simulink model "lab4_test2"  (R2016b)
settings: Solver=VariableStepAuto  StartTime=0.0  StopTime=totaltime  RelTol=1e-3
undefined symbols (not defined in the file or in its folder): h, st
libraries: xbsIndex_r4 x885
(part 2 of 2)

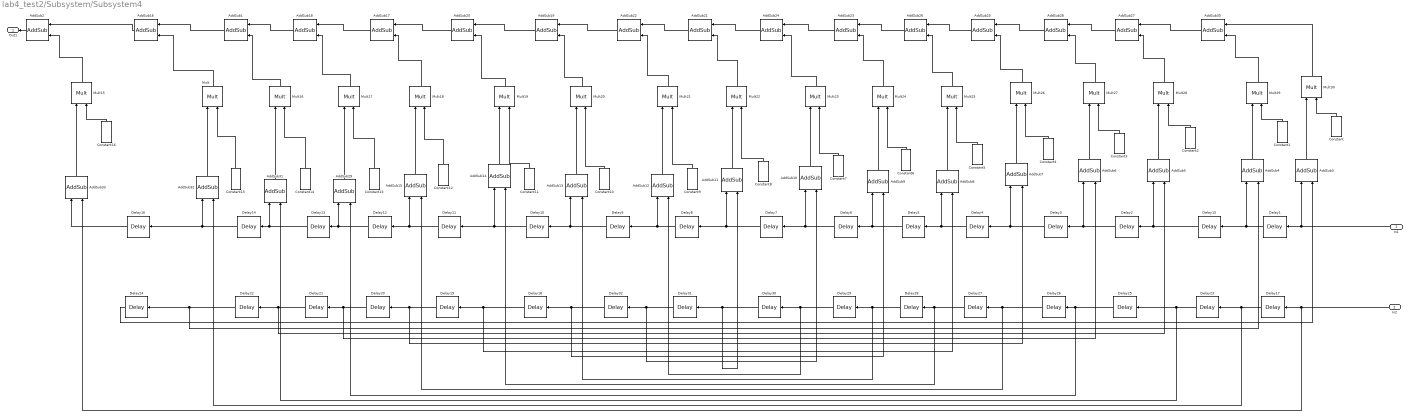
== system lab4_test2/Subsystem/Subsystem4 ==
  In1 : Inport
  In2 : Inport  Port=2
  AddSub{1..33} (33 alike) : xbsIndex_r4/AddSub  mode=Addition  use_carryin=off  use_carryout=off  en=off  latency=0  precision=User Defined  arith_type="Signed  (2's comp)"  n_bits=W  bin_pt=B  quantization=Truncate  overflow=Wrap  use_behavioral_HDL=off  hw_selection=Fabric  pipelined=off  dbl_ovrd=off  block_type=addsub
  Constant : xbsIndex_r4/Constant  const=h(1,10)  gui_display_data_type=Fixed-point  arith_type=Signed (2's comp)  n_bits=W  bin_pt=B  preci_type=Single  exp_width=8  frac_width=24  explicit_period=off  period=1  equ=P=C  opselect=C  inp2=PCIN>>17  opr=+  inp1=P  carry=CIN  dbl_ovrd=off  block_type=constant
  Constant1 : xbsIndex_r4/Constant  const=h(2,10)  gui_display_data_type=Fixed-point  arith_type=Signed (2's comp)  n_bits=W  bin_pt=B  preci_type=Single  exp_width=8  frac_width=24  explicit_period=off  period=1  equ=P=C  opselect=C  inp2=PCIN>>17  opr=+  inp1=P  carry=CIN  dbl_ovrd=off  block_type=constant
  Constant10 : xbsIndex_r4/Constant  const=h(11,10)  gui_display_data_type=Fixed-point  arith_type=Signed (2's comp)  n_bits=W  bin_pt=B  preci_type=Single  exp_width=8  frac_width=24  explicit_period=off  period=1  equ=P=C  opselect=C  inp2=PCIN>>17  opr=+  inp1=P  carry=CIN  dbl_ovrd=off  block_type=constant
  Constant11 : xbsIndex_r4/Constant  const=h(12,10)  gui_display_data_type=Fixed-point  arith_type=Signed (2's comp)  n_bits=W  bin_pt=B  preci_type=Single  exp_width=8  frac_width=24  explicit_period=off  period=1  equ=P=C  opselect=C  inp2=PCIN>>17  opr=+  inp1=P  carry=CIN  dbl_ovrd=off  block_type=constant
  Constant12 : xbsIndex_r4/Constant  const=h(13,10)  gui_display_data_type=Fixed-point  arith_type=Signed (2's comp)  n_bits=W  bin_pt=B  preci_type=Single  exp_width=8  frac_width=24  explicit_period=off  period=1  equ=P=C  opselect=C  inp2=PCIN>>17  opr=+  inp1=P  carry=CIN  dbl_ovrd=off  block_type=constant
  Constant13 : xbsIndex_r4/Constant  const=h(14,10)  gui_display_data_type=Fixed-point  arith_type=Signed (2's comp)  n_bits=W  bin_pt=B  preci_type=Single  exp_width=8  frac_width=24  explicit_period=off  period=1  equ=P=C  opselect=C  inp2=PCIN>>17  opr=+  inp1=P  carry=CIN  dbl_ovrd=off  block_type=constant
  Constant14 : xbsIndex_r4/Constant  const=h(15,10)  gui_display_data_type=Fixed-point  arith_type=Signed (2's comp)  n_bits=W  bin_pt=B  preci_type=Single  exp_width=8  frac_width=24  explicit_period=off  period=1  equ=P=C  opselect=C  inp2=PCIN>>17  opr=+  inp1=P  carry=CIN  dbl_ovrd=off  block_type=constant
  Constant15 : xbsIndex_r4/Constant  const=h(16,10)  gui_display_data_type=Fixed-point  arith_type=Signed (2's comp)  n_bits=W  bin_pt=B  preci_type=Single  exp_width=8  frac_width=24  explicit_period=off  period=1  equ=P=C  opselect=C  inp2=PCIN>>17  opr=+  inp1=P  carry=CIN  dbl_ovrd=off  block_type=constant
  Constant16 : xbsIndex_r4/Constant  const=h(17,10)  gui_display_data_type=Fixed-point  arith_type=Signed (2's comp)  n_bits=W  bin_pt=B  preci_type=Single  exp_width=8  frac_width=24  explicit_period=off  period=1  equ=P=C  opselect=C  inp2=PCIN>>17  opr=+  inp1=P  carry=CIN  dbl_ovrd=off  block_type=constant
  Constant2 : xbsIndex_r4/Constant  const=h(3,10)  gui_display_data_type=Fixed-point  arith_type=Signed (2's comp)  n_bits=W  bin_pt=B  preci_type=Single  exp_width=8  frac_width=24  explicit_period=off  period=1  equ=P=C  opselect=C  inp2=PCIN>>17  opr=+  inp1=P  carry=CIN  dbl_ovrd=off  block_type=constant
  Constant3 : xbsIndex_r4/Constant  const=h(4,10)  gui_display_data_type=Fixed-point  arith_type=Signed (2's comp)  n_bits=W  bin_pt=B  preci_type=Single  exp_width=8  frac_width=24  explicit_period=off  period=1  equ=P=C  opselect=C  inp2=PCIN>>17  opr=+  inp1=P  carry=CIN  dbl_ovrd=off  block_type=constant
  Constant4 : xbsIndex_r4/Constant  const=h(5,10)  gui_display_data_type=Fixed-point  arith_type=Signed (2's comp)  n_bits=W  bin_pt=B  preci_type=Single  exp_width=8  frac_width=24  explicit_period=off  period=1  equ=P=C  opselect=C  inp2=PCIN>>17  opr=+  inp1=P  carry=CIN  dbl_ovrd=off  block_type=constant
  Constant5 : xbsIndex_r4/Constant  const=h(6,10)  gui_display_data_type=Fixed-point  arith_type=Signed (2's comp)  n_bits=W  bin_pt=B  preci_type=Single  exp_width=8  frac_width=24  explicit_period=off  period=1  equ=P=C  opselect=C  inp2=PCIN>>17  opr=+  inp1=P  carry=CIN  dbl_ovrd=off  block_type=constant
  Constant6 : xbsIndex_r4/Constant  const=h(7,10)  gui_display_data_type=Fixed-point  arith_type=Signed (2's comp)  n_bits=W  bin_pt=B  preci_type=Single  exp_width=8  frac_width=24  explicit_period=off  period=1  equ=P=C  opselect=C  inp2=PCIN>>17  opr=+  inp1=P  carry=CIN  dbl_ovrd=off  block_type=constant
  Constant7 : xbsIndex_r4/Constant  const=h(8,10)  gui_display_data_type=Fixed-point  arith_type=Signed (2's comp)  n_bits=W  bin_pt=B  preci_type=Single  exp_width=8  frac_width=24  explicit_period=off  period=1  equ=P=C  opselect=C  inp2=PCIN>>17  opr=+  inp1=P  carry=CIN  dbl_ovrd=off  block_type=constant
  Constant8 : xbsIndex_r4/Constant  const=h(9,10)  gui_display_data_type=Fixed-point  arith_type=Signed (2's comp)  n_bits=W  bin_pt=B  preci_type=Single  exp_width=8  frac_width=24  explicit_period=off  period=1  equ=P=C  opselect=C  inp2=PCIN>>17  opr=+  inp1=P  carry=CIN  dbl_ovrd=off  block_type=constant
  Constant9 : xbsIndex_r4/Constant  const=h(10,10)  gui_display_data_type=Fixed-point  arith_type=Signed (2's comp)  n_bits=W  bin_pt=B  preci_type=Single  exp_width=8  frac_width=24  explicit_period=off  period=1  equ=P=C  opselect=C  inp2=PCIN>>17  opr=+  inp1=P  carry=CIN  dbl_ovrd=off  block_type=constant
  Delay{1..32} (32 alike) : xbsIndex_r4/Delay  rst=off  infoeditControl=Selection of Reset will increase slice count due to use of real FFs and instead of SRLs  en=off  latency=1  reg_retiming=off  dbl_ovrd=off  block_type=delay
  Mult{,15..30} (17 alike) : xbsIndex_r4/Mult  precision=User Defined  arith_type="Signed  (2's comp)"  n_bits=W  bin_pt=B  quantization="Round  (unbiased: +/- Inf)"  overflow=Flag as error  en=off  latency=0  use_behavioral_HDL=off  opt=Speed  use_embedded=on  optimum_pipeline=off  pipeline=on  dbl_ovrd=off  use_rpm=on  placement_style=Triangular  block_type=mult
  Out1 : Outport
  wires:
  AddSub2/1 -> Out1/1
  Constant14/1 -> Mult16/2
  Mult/1 -> AddSub16/2
  Mult16/1 -> AddSub1/2
  Constant15/1 -> Mult/2
  Constant13/1 -> Mult17/2
  Mult17/1 -> AddSub18/2
  Constant12/1 -> Mult18/2
  Constant11/1 -> Mult19/2
  Mult19/1 -> AddSub20/2
  Constant10/1 -> Mult20/2
  Mult20/1 -> AddSub19/2
  Constant9/1 -> Mult21/2
  Mult21/1 -> AddSub22/2
  Constant8/1 -> Mult22/2
  Constant7/1 -> Mult23/2
  Mult23/1 -> AddSub24/2
  Constant6/1 -> Mult24/2
  Constant5/1 -> Mult25/2
  Mult25/1 -> AddSub26/2
  Constant4/1 -> Mult26/2
  Mult26/1 -> AddSub25/2
  Constant3/1 -> Mult27/2
  Mult27/1 -> AddSub28/2
  Constant2/1 -> Mult28/2
  Constant1/1 -> Mult29/2
  Mult29/1 -> AddSub30/2
  Constant/1 -> Mult30/2
  AddSub1/1 -> AddSub16/1
  AddSub18/1 -> AddSub1/1
  AddSub17/1 -> AddSub18/1
  AddSub19/1 -> AddSub20/1
  AddSub22/1 -> AddSub19/1
  AddSub21/1 -> AddSub22/1
  AddSub23/1 -> AddSub24/1
  AddSub25/1 -> AddSub26/1
  AddSub28/1 -> AddSub25/1
  AddSub27/1 -> AddSub28/1
  Mult30/1 -> AddSub30/1
  Constant16/1 -> Mult15/2
  Mult15/1 -> AddSub2/2
  AddSub16/1 -> AddSub2/1
  AddSub20/1 -> AddSub17/1
  Mult18/1 -> AddSub17/2
  AddSub24/1 -> AddSub21/1
  Mult22/1 -> AddSub21/2
  AddSub26/1 -> AddSub23/1
  Mult24/1 -> AddSub23/2
  AddSub30/1 -> AddSub27/1
  Mult28/1 -> AddSub27/2
  In1/1 -> AddSub3/1, Delay1/1
  Delay1/1 -> AddSub4/1, Delay15/1
  Delay15/1 -> AddSub5/1, Delay2/1
  Delay2/1 -> AddSub6/1, Delay3/1
  Delay3/1 -> AddSub7/1, Delay4/1
  Delay4/1 -> AddSub8/1, Delay5/1
  Delay5/1 -> AddSub9/1, Delay6/1
  Delay6/1 -> AddSub10/1, Delay7/1
  Delay7/1 -> AddSub11/1, Delay8/1
  Delay8/1 -> AddSub12/1, Delay9/1
  Delay9/1 -> AddSub13/1, Delay10/1
  Delay10/1 -> AddSub14/1, Delay11/1
  Delay11/1 -> AddSub15/1, Delay12/1
  Delay12/1 -> AddSub29/1, Delay13/1
  Delay13/1 -> AddSub31/1, Delay14/1
  Delay14/1 -> AddSub32/1, Delay16/1
  In2/1 -> AddSub33/2, Delay17/1
  Delay17/1 -> AddSub32/2, Delay23/1
  Delay23/1 -> AddSub31/2, Delay25/1
  Delay25/1 -> AddSub29/2, Delay26/1
  Delay26/1 -> AddSub15/2, Delay27/1
  Delay27/1 -> AddSub14/2, Delay28/1
  Delay28/1 -> AddSub13/2, Delay29/1
  Delay29/1 -> AddSub12/2, Delay30/1
  Delay30/1 -> AddSub11/2, Delay31/1
  Delay31/1 -> AddSub10/2, Delay32/1
  Delay32/1 -> AddSub9/2, Delay18/1
  Delay18/1 -> AddSub8/2, Delay19/1
  Delay19/1 -> AddSub7/2, Delay20/1
  Delay20/1 -> AddSub6/2, Delay21/1
  Delay21/1 -> AddSub5/2, Delay22/1
  Delay22/1 -> AddSub4/2, Delay24/1
  AddSub3/1 -> Mult30/1
  Delay16/1 -> AddSub33/1
  AddSub33/1 -> Mult15/1
  AddSub32/1 -> Mult/1
  AddSub31/1 -> Mult16/1
  AddSub29/1 -> Mult17/1
  AddSub15/1 -> Mult18/1
  AddSub14/1 -> Mult19/1
  AddSub13/1 -> Mult20/1
  AddSub12/1 -> Mult21/1
  AddSub11/1 -> Mult22/1
  AddSub10/1 -> Mult23/1
  AddSub9/1 -> Mult24/1
  AddSub8/1 -> Mult25/1
  AddSub7/1 -> Mult26/1
  AddSub6/1 -> Mult27/1
  AddSub5/1 -> Mult28/1
  AddSub4/1 -> Mult29/1
  Delay24/1 -> AddSub3/2

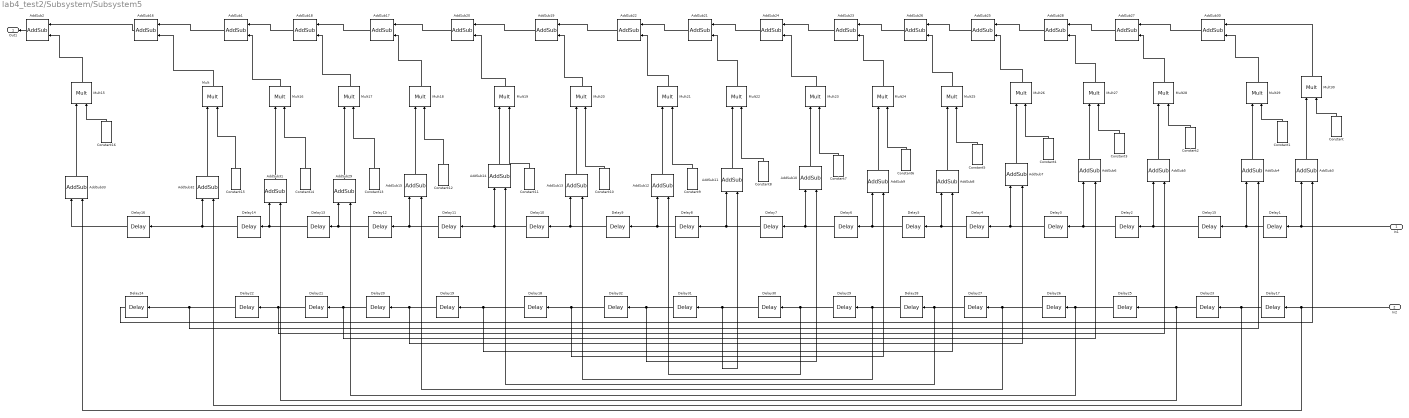
== system lab4_test2/Subsystem/Subsystem5 ==
  In1 : Inport
  In2 : Inport  Port=2
  AddSub{1..33} (33 alike) : xbsIndex_r4/AddSub  mode=Addition  use_carryin=off  use_carryout=off  en=off  latency=0  precision=User Defined  arith_type="Signed  (2's comp)"  n_bits=W  bin_pt=B  quantization=Truncate  overflow=Wrap  use_behavioral_HDL=off  hw_selection=Fabric  pipelined=off  dbl_ovrd=off  block_type=addsub
  Constant : xbsIndex_r4/Constant  const=h(1,13)  gui_display_data_type=Fixed-point  arith_type=Signed (2's comp)  n_bits=W  bin_pt=B  preci_type=Single  exp_width=8  frac_width=24  explicit_period=off  period=1  equ=P=C  opselect=C  inp2=PCIN>>17  opr=+  inp1=P  carry=CIN  dbl_ovrd=off  block_type=constant
  Constant1 : xbsIndex_r4/Constant  const=h(2,13)  gui_display_data_type=Fixed-point  arith_type=Signed (2's comp)  n_bits=W  bin_pt=B  preci_type=Single  exp_width=8  frac_width=24  explicit_period=off  period=1  equ=P=C  opselect=C  inp2=PCIN>>17  opr=+  inp1=P  carry=CIN  dbl_ovrd=off  block_type=constant
  Constant10 : xbsIndex_r4/Constant  const=h(11,13)  gui_display_data_type=Fixed-point  arith_type=Signed (2's comp)  n_bits=W  bin_pt=B  preci_type=Single  exp_width=8  frac_width=24  explicit_period=off  period=1  equ=P=C  opselect=C  inp2=PCIN>>17  opr=+  inp1=P  carry=CIN  dbl_ovrd=off  block_type=constant
  Constant11 : xbsIndex_r4/Constant  const=h(12,13)  gui_display_data_type=Fixed-point  arith_type=Signed (2's comp)  n_bits=W  bin_pt=B  preci_type=Single  exp_width=8  frac_width=24  explicit_period=off  period=1  equ=P=C  opselect=C  inp2=PCIN>>17  opr=+  inp1=P  carry=CIN  dbl_ovrd=off  block_type=constant
  Constant12 : xbsIndex_r4/Constant  const=h(13,13)  gui_display_data_type=Fixed-point  arith_type=Signed (2's comp)  n_bits=W  bin_pt=B  preci_type=Single  exp_width=8  frac_width=24  explicit_period=off  period=1  equ=P=C  opselect=C  inp2=PCIN>>17  opr=+  inp1=P  carry=CIN  dbl_ovrd=off  block_type=constant
  Constant13 : xbsIndex_r4/Constant  const=h(14,13)  gui_display_data_type=Fixed-point  arith_type=Signed (2's comp)  n_bits=W  bin_pt=B  preci_type=Single  exp_width=8  frac_width=24  explicit_period=off  period=1  equ=P=C  opselect=C  inp2=PCIN>>17  opr=+  inp1=P  carry=CIN  dbl_ovrd=off  block_type=constant
  Constant14 : xbsIndex_r4/Constant  const=h(15,13)  gui_display_data_type=Fixed-point  arith_type=Signed (2's comp)  n_bits=W  bin_pt=B  preci_type=Single  exp_width=8  frac_width=24  explicit_period=off  period=1  equ=P=C  opselect=C  inp2=PCIN>>17  opr=+  inp1=P  carry=CIN  dbl_ovrd=off  block_type=constant
  Constant15 : xbsIndex_r4/Constant  const=h(16,13)  gui_display_data_type=Fixed-point  arith_type=Signed (2's comp)  n_bits=W  bin_pt=B  preci_type=Single  exp_width=8  frac_width=24  explicit_period=off  period=1  equ=P=C  opselect=C  inp2=PCIN>>17  opr=+  inp1=P  carry=CIN  dbl_ovrd=off  block_type=constant
  Constant16 : xbsIndex_r4/Constant  const=h(17,13)  gui_display_data_type=Fixed-point  arith_type=Signed (2's comp)  n_bits=W  bin_pt=B  preci_type=Single  exp_width=8  frac_width=24  explicit_period=off  period=1  equ=P=C  opselect=C  inp2=PCIN>>17  opr=+  inp1=P  carry=CIN  dbl_ovrd=off  block_type=constant
  Constant2 : xbsIndex_r4/Constant  const=h(3,13)  gui_display_data_type=Fixed-point  arith_type=Signed (2's comp)  n_bits=W  bin_pt=B  preci_type=Single  exp_width=8  frac_width=24  explicit_period=off  period=1  equ=P=C  opselect=C  inp2=PCIN>>17  opr=+  inp1=P  carry=CIN  dbl_ovrd=off  block_type=constant
  Constant3 : xbsIndex_r4/Constant  const=h(4,13)  gui_display_data_type=Fixed-point  arith_type=Signed (2's comp)  n_bits=W  bin_pt=B  preci_type=Single  exp_width=8  frac_width=24  explicit_period=off  period=1  equ=P=C  opselect=C  inp2=PCIN>>17  opr=+  inp1=P  carry=CIN  dbl_ovrd=off  block_type=constant
  Constant4 : xbsIndex_r4/Constant  const=h(5,13)  gui_display_data_type=Fixed-point  arith_type=Signed (2's comp)  n_bits=W  bin_pt=B  preci_type=Single  exp_width=8  frac_width=24  explicit_period=off  period=1  equ=P=C  opselect=C  inp2=PCIN>>17  opr=+  inp1=P  carry=CIN  dbl_ovrd=off  block_type=constant
  Constant5 : xbsIndex_r4/Constant  const=h(6,13)  gui_display_data_type=Fixed-point  arith_type=Signed (2's comp)  n_bits=W  bin_pt=B  preci_type=Single  exp_width=8  frac_width=24  explicit_period=off  period=1  equ=P=C  opselect=C  inp2=PCIN>>17  opr=+  inp1=P  carry=CIN  dbl_ovrd=off  block_type=constant
  Constant6 : xbsIndex_r4/Constant  const=h(7,13)  gui_display_data_type=Fixed-point  arith_type=Signed (2's comp)  n_bits=W  bin_pt=B  preci_type=Single  exp_width=8  frac_width=24  explicit_period=off  period=1  equ=P=C  opselect=C  inp2=PCIN>>17  opr=+  inp1=P  carry=CIN  dbl_ovrd=off  block_type=constant
  Constant7 : xbsIndex_r4/Constant  const=h(8,13)  gui_display_data_type=Fixed-point  arith_type=Signed (2's comp)  n_bits=W  bin_pt=B  preci_type=Single  exp_width=8  frac_width=24  explicit_period=off  period=1  equ=P=C  opselect=C  inp2=PCIN>>17  opr=+  inp1=P  carry=CIN  dbl_ovrd=off  block_type=constant
  Constant8 : xbsIndex_r4/Constant  const=h(9,13)  gui_display_data_type=Fixed-point  arith_type=Signed (2's comp)  n_bits=W  bin_pt=B  preci_type=Single  exp_width=8  frac_width=24  explicit_period=off  period=1  equ=P=C  opselect=C  inp2=PCIN>>17  opr=+  inp1=P  carry=CIN  dbl_ovrd=off  block_type=constant
  Constant9 : xbsIndex_r4/Constant  const=h(10,13)  gui_display_data_type=Fixed-point  arith_type=Signed (2's comp)  n_bits=W  bin_pt=B  preci_type=Single  exp_width=8  frac_width=24  explicit_period=off  period=1  equ=P=C  opselect=C  inp2=PCIN>>17  opr=+  inp1=P  carry=CIN  dbl_ovrd=off  block_type=constant
  Delay{1..32} (32 alike) : xbsIndex_r4/Delay  rst=off  infoeditControl=Selection of Reset will increase slice count due to use of real FFs and instead of SRLs  en=off  latency=1  reg_retiming=off  dbl_ovrd=off  block_type=delay
  Mult{,15..30} (17 alike) : xbsIndex_r4/Mult  precision=User Defined  arith_type="Signed  (2's comp)"  n_bits=W  bin_pt=B  quantization="Round  (unbiased: +/- Inf)"  overflow=Flag as error  en=off  latency=0  use_behavioral_HDL=off  opt=Speed  use_embedded=on  optimum_pipeline=off  pipeline=on  dbl_ovrd=off  use_rpm=on  placement_style=Triangular  block_type=mult
  Out1 : Outport
  wires:
  AddSub2/1 -> Out1/1
  Constant14/1 -> Mult16/2
  Mult/1 -> AddSub16/2
  Mult16/1 -> AddSub1/2
  Constant15/1 -> Mult/2
  Constant13/1 -> Mult17/2
  Mult17/1 -> AddSub18/2
  Constant12/1 -> Mult18/2
  Constant11/1 -> Mult19/2
  Mult19/1 -> AddSub20/2
  Constant10/1 -> Mult20/2
  Mult20/1 -> AddSub19/2
  Constant9/1 -> Mult21/2
  Mult21/1 -> AddSub22/2
  Constant8/1 -> Mult22/2
  Constant7/1 -> Mult23/2
  Mult23/1 -> AddSub24/2
  Constant6/1 -> Mult24/2
  Constant5/1 -> Mult25/2
  Mult25/1 -> AddSub26/2
  Constant4/1 -> Mult26/2
  Mult26/1 -> AddSub25/2
  Constant3/1 -> Mult27/2
  Mult27/1 -> AddSub28/2
  Constant2/1 -> Mult28/2
  Constant1/1 -> Mult29/2
  Mult29/1 -> AddSub30/2
  Constant/1 -> Mult30/2
  AddSub1/1 -> AddSub16/1
  AddSub18/1 -> AddSub1/1
  AddSub17/1 -> AddSub18/1
  AddSub19/1 -> AddSub20/1
  AddSub22/1 -> AddSub19/1
  AddSub21/1 -> AddSub22/1
  AddSub23/1 -> AddSub24/1
  AddSub25/1 -> AddSub26/1
  AddSub28/1 -> AddSub25/1
  AddSub27/1 -> AddSub28/1
  Mult30/1 -> AddSub30/1
  Constant16/1 -> Mult15/2
  Mult15/1 -> AddSub2/2
  AddSub16/1 -> AddSub2/1
  AddSub20/1 -> AddSub17/1
  Mult18/1 -> AddSub17/2
  AddSub24/1 -> AddSub21/1
  Mult22/1 -> AddSub21/2
  AddSub26/1 -> AddSub23/1
  Mult24/1 -> AddSub23/2
  AddSub30/1 -> AddSub27/1
  Mult28/1 -> AddSub27/2
  In1/1 -> AddSub3/1, Delay1/1
  Delay1/1 -> AddSub4/1, Delay15/1
  Delay15/1 -> AddSub5/1, Delay2/1
  Delay2/1 -> AddSub6/1, Delay3/1
  Delay3/1 -> AddSub7/1, Delay4/1
  Delay4/1 -> AddSub8/1, Delay5/1
  Delay5/1 -> AddSub9/1, Delay6/1
  Delay6/1 -> AddSub10/1, Delay7/1
  Delay7/1 -> AddSub11/1, Delay8/1
  Delay8/1 -> AddSub12/1, Delay9/1
  Delay9/1 -> AddSub13/1, Delay10/1
  Delay10/1 -> AddSub14/1, Delay11/1
  Delay11/1 -> AddSub15/1, Delay12/1
  Delay12/1 -> AddSub29/1, Delay13/1
  Delay13/1 -> AddSub31/1, Delay14/1
  Delay14/1 -> AddSub32/1, Delay16/1
  In2/1 -> AddSub33/2, Delay17/1
  Delay17/1 -> AddSub32/2, Delay23/1
  Delay23/1 -> AddSub31/2, Delay25/1
  Delay25/1 -> AddSub29/2, Delay26/1
  Delay26/1 -> AddSub15/2, Delay27/1
  Delay27/1 -> AddSub14/2, Delay28/1
  Delay28/1 -> AddSub13/2, Delay29/1
  Delay29/1 -> AddSub12/2, Delay30/1
  Delay30/1 -> AddSub11/2, Delay31/1
  Delay31/1 -> AddSub10/2, Delay32/1
  Delay32/1 -> AddSub9/2, Delay18/1
  Delay18/1 -> AddSub8/2, Delay19/1
  Delay19/1 -> AddSub7/2, Delay20/1
  Delay20/1 -> AddSub6/2, Delay21/1
  Delay21/1 -> AddSub5/2, Delay22/1
  Delay22/1 -> AddSub4/2, Delay24/1
  AddSub3/1 -> Mult30/1
  Delay16/1 -> AddSub33/1
  AddSub33/1 -> Mult15/1
  AddSub32/1 -> Mult/1
  AddSub31/1 -> Mult16/1
  AddSub29/1 -> Mult17/1
  AddSub15/1 -> Mult18/1
  AddSub14/1 -> Mult19/1
  AddSub13/1 -> Mult20/1
  AddSub12/1 -> Mult21/1
  AddSub11/1 -> Mult22/1
  AddSub10/1 -> Mult23/1
  AddSub9/1 -> Mult24/1
  AddSub8/1 -> Mult25/1
  AddSub7/1 -> Mult26/1
  AddSub6/1 -> Mult27/1
  AddSub5/1 -> Mult28/1
  AddSub4/1 -> Mult29/1
  Delay24/1 -> AddSub3/2

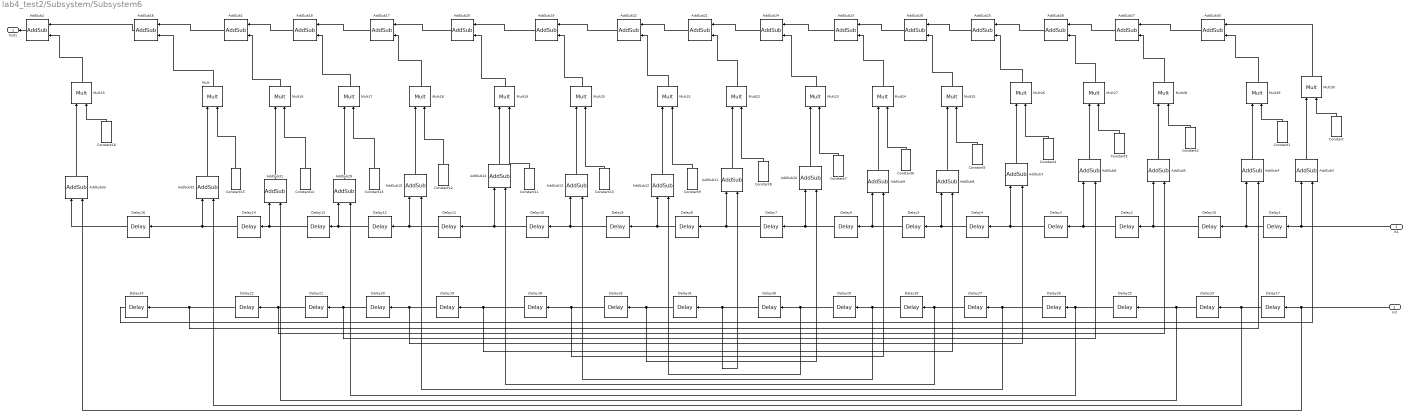
== system lab4_test2/Subsystem/Subsystem6 ==
  In1 : Inport
  In2 : Inport  Port=2
  AddSub{1..33} (33 alike) : xbsIndex_r4/AddSub  mode=Addition  use_carryin=off  use_carryout=off  en=off  latency=0  precision=User Defined  arith_type="Signed  (2's comp)"  n_bits=W  bin_pt=B  quantization=Truncate  overflow=Wrap  use_behavioral_HDL=off  hw_selection=Fabric  pipelined=off  dbl_ovrd=off  block_type=addsub
  Constant : xbsIndex_r4/Constant  const=h(1,12)  gui_display_data_type=Fixed-point  arith_type=Signed (2's comp)  n_bits=W  bin_pt=B  preci_type=Single  exp_width=8  frac_width=24  explicit_period=off  period=1  equ=P=C  opselect=C  inp2=PCIN>>17  opr=+  inp1=P  carry=CIN  dbl_ovrd=off  block_type=constant
  Constant1 : xbsIndex_r4/Constant  const=h(2,12)  gui_display_data_type=Fixed-point  arith_type=Signed (2's comp)  n_bits=W  bin_pt=B  preci_type=Single  exp_width=8  frac_width=24  explicit_period=off  period=1  equ=P=C  opselect=C  inp2=PCIN>>17  opr=+  inp1=P  carry=CIN  dbl_ovrd=off  block_type=constant
  Constant10 : xbsIndex_r4/Constant  const=h(11,12)  gui_display_data_type=Fixed-point  arith_type=Signed (2's comp)  n_bits=W  bin_pt=B  preci_type=Single  exp_width=8  frac_width=24  explicit_period=off  period=1  equ=P=C  opselect=C  inp2=PCIN>>17  opr=+  inp1=P  carry=CIN  dbl_ovrd=off  block_type=constant
  Constant11 : xbsIndex_r4/Constant  const=h(12,12)  gui_display_data_type=Fixed-point  arith_type=Signed (2's comp)  n_bits=W  bin_pt=B  preci_type=Single  exp_width=8  frac_width=24  explicit_period=off  period=1  equ=P=C  opselect=C  inp2=PCIN>>17  opr=+  inp1=P  carry=CIN  dbl_ovrd=off  block_type=constant
  Constant12 : xbsIndex_r4/Constant  const=h(13,12)  gui_display_data_type=Fixed-point  arith_type=Signed (2's comp)  n_bits=W  bin_pt=B  preci_type=Single  exp_width=8  frac_width=24  explicit_period=off  period=1  equ=P=C  opselect=C  inp2=PCIN>>17  opr=+  inp1=P  carry=CIN  dbl_ovrd=off  block_type=constant
  Constant13 : xbsIndex_r4/Constant  const=h(14,12)  gui_display_data_type=Fixed-point  arith_type=Signed (2's comp)  n_bits=W  bin_pt=B  preci_type=Single  exp_width=8  frac_width=24  explicit_period=off  period=1  equ=P=C  opselect=C  inp2=PCIN>>17  opr=+  inp1=P  carry=CIN  dbl_ovrd=off  block_type=constant
  Constant14 : xbsIndex_r4/Constant  const=h(15,12)  gui_display_data_type=Fixed-point  arith_type=Signed (2's comp)  n_bits=W  bin_pt=B  preci_type=Single  exp_width=8  frac_width=24  explicit_period=off  period=1  equ=P=C  opselect=C  inp2=PCIN>>17  opr=+  inp1=P  carry=CIN  dbl_ovrd=off  block_type=constant
  Constant15 : xbsIndex_r4/Constant  const=h(16,12)  gui_display_data_type=Fixed-point  arith_type=Signed (2's comp)  n_bits=W  bin_pt=B  preci_type=Single  exp_width=8  frac_width=24  explicit_period=off  period=1  equ=P=C  opselect=C  inp2=PCIN>>17  opr=+  inp1=P  carry=CIN  dbl_ovrd=off  block_type=constant
  Constant16 : xbsIndex_r4/Constant  const=h(17,12)  gui_display_data_type=Fixed-point  arith_type=Signed (2's comp)  n_bits=W  bin_pt=B  preci_type=Single  exp_width=8  frac_width=24  explicit_period=off  period=1  equ=P=C  opselect=C  inp2=PCIN>>17  opr=+  inp1=P  carry=CIN  dbl_ovrd=off  block_type=constant
  Constant2 : xbsIndex_r4/Constant  const=h(3,12)  gui_display_data_type=Fixed-point  arith_type=Signed (2's comp)  n_bits=W  bin_pt=B  preci_type=Single  exp_width=8  frac_width=24  explicit_period=off  period=1  equ=P=C  opselect=C  inp2=PCIN>>17  opr=+  inp1=P  carry=CIN  dbl_ovrd=off  block_type=constant
  Constant3 : xbsIndex_r4/Constant  const=h(4,12)  gui_display_data_type=Fixed-point  arith_type=Signed (2's comp)  n_bits=W  bin_pt=B  preci_type=Single  exp_width=8  frac_width=24  explicit_period=off  period=1  equ=P=C  opselect=C  inp2=PCIN>>17  opr=+  inp1=P  carry=CIN  dbl_ovrd=off  block_type=constant
  Constant4 : xbsIndex_r4/Constant  const=h(5,12)  gui_display_data_type=Fixed-point  arith_type=Signed (2's comp)  n_bits=W  bin_pt=B  preci_type=Single  exp_width=8  frac_width=24  explicit_period=off  period=1  equ=P=C  opselect=C  inp2=PCIN>>17  opr=+  inp1=P  carry=CIN  dbl_ovrd=off  block_type=constant
  Constant5 : xbsIndex_r4/Constant  const=h(6,12)  gui_display_data_type=Fixed-point  arith_type=Signed (2's comp)  n_bits=W  bin_pt=B  preci_type=Single  exp_width=8  frac_width=24  explicit_period=off  period=1  equ=P=C  opselect=C  inp2=PCIN>>17  opr=+  inp1=P  carry=CIN  dbl_ovrd=off  block_type=constant
  Constant6 : xbsIndex_r4/Constant  const=h(7,12)  gui_display_data_type=Fixed-point  arith_type=Signed (2's comp)  n_bits=W  bin_pt=B  preci_type=Single  exp_width=8  frac_width=24  explicit_period=off  period=1  equ=P=C  opselect=C  inp2=PCIN>>17  opr=+  inp1=P  carry=CIN  dbl_ovrd=off  block_type=constant
  Constant7 : xbsIndex_r4/Constant  const=h(8,12)  gui_display_data_type=Fixed-point  arith_type=Signed (2's comp)  n_bits=W  bin_pt=B  preci_type=Single  exp_width=8  frac_width=24  explicit_period=off  period=1  equ=P=C  opselect=C  inp2=PCIN>>17  opr=+  inp1=P  carry=CIN  dbl_ovrd=off  block_type=constant
  Constant8 : xbsIndex_r4/Constant  const=h(9,12)  gui_display_data_type=Fixed-point  arith_type=Signed (2's comp)  n_bits=W  bin_pt=B  preci_type=Single  exp_width=8  frac_width=24  explicit_period=off  period=1  equ=P=C  opselect=C  inp2=PCIN>>17  opr=+  inp1=P  carry=CIN  dbl_ovrd=off  block_type=constant
  Constant9 : xbsIndex_r4/Constant  const=h(10,12)  gui_display_data_type=Fixed-point  arith_type=Signed (2's comp)  n_bits=W  bin_pt=B  preci_type=Single  exp_width=8  frac_width=24  explicit_period=off  period=1  equ=P=C  opselect=C  inp2=PCIN>>17  opr=+  inp1=P  carry=CIN  dbl_ovrd=off  block_type=constant
  Delay{1..32} (32 alike) : xbsIndex_r4/Delay  rst=off  infoeditControl=Selection of Reset will increase slice count due to use of real FFs and instead of SRLs  en=off  latency=1  reg_retiming=off  dbl_ovrd=off  block_type=delay
  Mult{,15..30} (17 alike) : xbsIndex_r4/Mult  precision=User Defined  arith_type="Signed  (2's comp)"  n_bits=W  bin_pt=B  quantization="Round  (unbiased: +/- Inf)"  overflow=Flag as error  en=off  latency=0  use_behavioral_HDL=off  opt=Speed  use_embedded=on  optimum_pipeline=off  pipeline=on  dbl_ovrd=off  use_rpm=on  placement_style=Triangular  block_type=mult
  Out1 : Outport
  wires:
  AddSub2/1 -> Out1/1
  Constant14/1 -> Mult16/2
  Mult/1 -> AddSub16/2
  Mult16/1 -> AddSub1/2
  Constant15/1 -> Mult/2
  Constant13/1 -> Mult17/2
  Mult17/1 -> AddSub18/2
  Constant12/1 -> Mult18/2
  Constant11/1 -> Mult19/2
  Mult19/1 -> AddSub20/2
  Constant10/1 -> Mult20/2
  Mult20/1 -> AddSub19/2
  Constant9/1 -> Mult21/2
  Mult21/1 -> AddSub22/2
  Constant8/1 -> Mult22/2
  Constant7/1 -> Mult23/2
  Mult23/1 -> AddSub24/2
  Constant6/1 -> Mult24/2
  Constant5/1 -> Mult25/2
  Mult25/1 -> AddSub26/2
  Constant4/1 -> Mult26/2
  Mult26/1 -> AddSub25/2
  Constant3/1 -> Mult27/2
  Mult27/1 -> AddSub28/2
  Constant2/1 -> Mult28/2
  Constant1/1 -> Mult29/2
  Mult29/1 -> AddSub30/2
  Constant/1 -> Mult30/2
  AddSub1/1 -> AddSub16/1
  AddSub18/1 -> AddSub1/1
  AddSub17/1 -> AddSub18/1
  AddSub19/1 -> AddSub20/1
  AddSub22/1 -> AddSub19/1
  AddSub21/1 -> AddSub22/1
  AddSub23/1 -> AddSub24/1
  AddSub25/1 -> AddSub26/1
  AddSub28/1 -> AddSub25/1
  AddSub27/1 -> AddSub28/1
  Mult30/1 -> AddSub30/1
  Constant16/1 -> Mult15/2
  Mult15/1 -> AddSub2/2
  AddSub16/1 -> AddSub2/1
  AddSub20/1 -> AddSub17/1
  Mult18/1 -> AddSub17/2
  AddSub24/1 -> AddSub21/1
  Mult22/1 -> AddSub21/2
  AddSub26/1 -> AddSub23/1
  Mult24/1 -> AddSub23/2
  AddSub30/1 -> AddSub27/1
  Mult28/1 -> AddSub27/2
  In1/1 -> AddSub3/1, Delay1/1
  Delay1/1 -> AddSub4/1, Delay15/1
  Delay15/1 -> AddSub5/1, Delay2/1
  Delay2/1 -> AddSub6/1, Delay3/1
  Delay3/1 -> AddSub7/1, Delay4/1
  Delay4/1 -> AddSub8/1, Delay5/1
  Delay5/1 -> AddSub9/1, Delay6/1
  Delay6/1 -> AddSub10/1, Delay7/1
  Delay7/1 -> AddSub11/1, Delay8/1
  Delay8/1 -> AddSub12/1, Delay9/1
  Delay9/1 -> AddSub13/1, Delay10/1
  Delay10/1 -> AddSub14/1, Delay11/1
  Delay11/1 -> AddSub15/1, Delay12/1
  Delay12/1 -> AddSub29/1, Delay13/1
  Delay13/1 -> AddSub31/1, Delay14/1
  Delay14/1 -> AddSub32/1, Delay16/1
  In2/1 -> AddSub33/2, Delay17/1
  Delay17/1 -> AddSub32/2, Delay23/1
  Delay23/1 -> AddSub31/2, Delay25/1
  Delay25/1 -> AddSub29/2, Delay26/1
  Delay26/1 -> AddSub15/2, Delay27/1
  Delay27/1 -> AddSub14/2, Delay28/1
  Delay28/1 -> AddSub13/2, Delay29/1
  Delay29/1 -> AddSub12/2, Delay30/1
  Delay30/1 -> AddSub11/2, Delay31/1
  Delay31/1 -> AddSub10/2, Delay32/1
  Delay32/1 -> AddSub9/2, Delay18/1
  Delay18/1 -> AddSub8/2, Delay19/1
  Delay19/1 -> AddSub7/2, Delay20/1
  Delay20/1 -> AddSub6/2, Delay21/1
  Delay21/1 -> AddSub5/2, Delay22/1
  Delay22/1 -> AddSub4/2, Delay24/1
  AddSub3/1 -> Mult30/1
  Delay16/1 -> AddSub33/1
  AddSub33/1 -> Mult15/1
  AddSub32/1 -> Mult/1
  AddSub31/1 -> Mult16/1
  AddSub29/1 -> Mult17/1
  AddSub15/1 -> Mult18/1
  AddSub14/1 -> Mult19/1
  AddSub13/1 -> Mult20/1
  AddSub12/1 -> Mult21/1
  AddSub11/1 -> Mult22/1
  AddSub10/1 -> Mult23/1
  AddSub9/1 -> Mult24/1
  AddSub8/1 -> Mult25/1
  AddSub7/1 -> Mult26/1
  AddSub6/1 -> Mult27/1
  AddSub5/1 -> Mult28/1
  AddSub4/1 -> Mult29/1
  Delay24/1 -> AddSub3/2

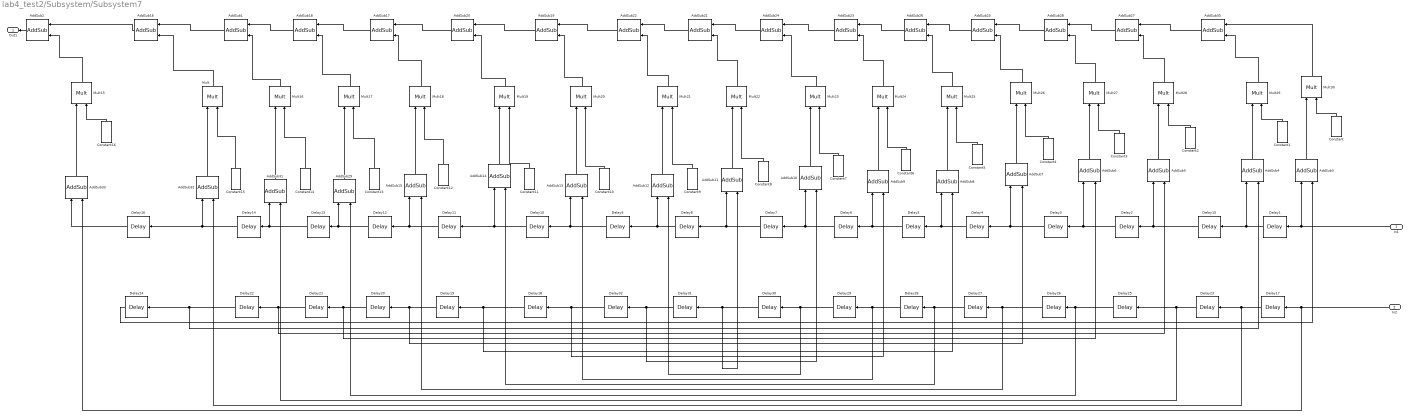
== system lab4_test2/Subsystem/Subsystem7 ==
  In1 : Inport
  In2 : Inport  Port=2
  AddSub{1..33} (33 alike) : xbsIndex_r4/AddSub  mode=Addition  use_carryin=off  use_carryout=off  en=off  latency=0  precision=User Defined  arith_type="Signed  (2's comp)"  n_bits=W  bin_pt=B  quantization=Truncate  overflow=Wrap  use_behavioral_HDL=off  hw_selection=Fabric  pipelined=off  dbl_ovrd=off  block_type=addsub
  Constant : xbsIndex_r4/Constant  const=h(1,11)  gui_display_data_type=Fixed-point  arith_type=Signed (2's comp)  n_bits=W  bin_pt=B  preci_type=Single  exp_width=8  frac_width=24  explicit_period=off  period=1  equ=P=C  opselect=C  inp2=PCIN>>17  opr=+  inp1=P  carry=CIN  dbl_ovrd=off  block_type=constant
  Constant1 : xbsIndex_r4/Constant  const=h(2,11)  gui_display_data_type=Fixed-point  arith_type=Signed (2's comp)  n_bits=W  bin_pt=B  preci_type=Single  exp_width=8  frac_width=24  explicit_period=off  period=1  equ=P=C  opselect=C  inp2=PCIN>>17  opr=+  inp1=P  carry=CIN  dbl_ovrd=off  block_type=constant
  Constant10 : xbsIndex_r4/Constant  const=h(11,11)  gui_display_data_type=Fixed-point  arith_type=Signed (2's comp)  n_bits=W  bin_pt=B  preci_type=Single  exp_width=8  frac_width=24  explicit_period=off  period=1  equ=P=C  opselect=C  inp2=PCIN>>17  opr=+  inp1=P  carry=CIN  dbl_ovrd=off  block_type=constant
  Constant11 : xbsIndex_r4/Constant  const=h(12,11)  gui_display_data_type=Fixed-point  arith_type=Signed (2's comp)  n_bits=W  bin_pt=B  preci_type=Single  exp_width=8  frac_width=24  explicit_period=off  period=1  equ=P=C  opselect=C  inp2=PCIN>>17  opr=+  inp1=P  carry=CIN  dbl_ovrd=off  block_type=constant
  Constant12 : xbsIndex_r4/Constant  const=h(13,11)  gui_display_data_type=Fixed-point  arith_type=Signed (2's comp)  n_bits=W  bin_pt=B  preci_type=Single  exp_width=8  frac_width=24  explicit_period=off  period=1  equ=P=C  opselect=C  inp2=PCIN>>17  opr=+  inp1=P  carry=CIN  dbl_ovrd=off  block_type=constant
  Constant13 : xbsIndex_r4/Constant  const=h(14,11)  gui_display_data_type=Fixed-point  arith_type=Signed (2's comp)  n_bits=W  bin_pt=B  preci_type=Single  exp_width=8  frac_width=24  explicit_period=off  period=1  equ=P=C  opselect=C  inp2=PCIN>>17  opr=+  inp1=P  carry=CIN  dbl_ovrd=off  block_type=constant
  Constant14 : xbsIndex_r4/Constant  const=h(15,11)  gui_display_data_type=Fixed-point  arith_type=Signed (2's comp)  n_bits=W  bin_pt=B  preci_type=Single  exp_width=8  frac_width=24  explicit_period=off  period=1  equ=P=C  opselect=C  inp2=PCIN>>17  opr=+  inp1=P  carry=CIN  dbl_ovrd=off  block_type=constant
  Constant15 : xbsIndex_r4/Constant  const=h(16,11)  gui_display_data_type=Fixed-point  arith_type=Signed (2's comp)  n_bits=W  bin_pt=B  preci_type=Single  exp_width=8  frac_width=24  explicit_period=off  period=1  equ=P=C  opselect=C  inp2=PCIN>>17  opr=+  inp1=P  carry=CIN  dbl_ovrd=off  block_type=constant
  Constant16 : xbsIndex_r4/Constant  const=h(17,11)  gui_display_data_type=Fixed-point  arith_type=Signed (2's comp)  n_bits=W  bin_pt=B  preci_type=Single  exp_width=8  frac_width=24  explicit_period=off  period=1  equ=P=C  opselect=C  inp2=PCIN>>17  opr=+  inp1=P  carry=CIN  dbl_ovrd=off  block_type=constant
  Constant2 : xbsIndex_r4/Constant  const=h(3,11)  gui_display_data_type=Fixed-point  arith_type=Signed (2's comp)  n_bits=W  bin_pt=B  preci_type=Single  exp_width=8  frac_width=24  explicit_period=off  period=1  equ=P=C  opselect=C  inp2=PCIN>>17  opr=+  inp1=P  carry=CIN  dbl_ovrd=off  block_type=constant
  Constant3 : xbsIndex_r4/Constant  const=h(4,11)  gui_display_data_type=Fixed-point  arith_type=Signed (2's comp)  n_bits=W  bin_pt=B  preci_type=Single  exp_width=8  frac_width=24  explicit_period=off  period=1  equ=P=C  opselect=C  inp2=PCIN>>17  opr=+  inp1=P  carry=CIN  dbl_ovrd=off  block_type=constant
  Constant4 : xbsIndex_r4/Constant  const=h(5,11)  gui_display_data_type=Fixed-point  arith_type=Signed (2's comp)  n_bits=W  bin_pt=B  preci_type=Single  exp_width=8  frac_width=24  explicit_period=off  period=1  equ=P=C  opselect=C  inp2=PCIN>>17  opr=+  inp1=P  carry=CIN  dbl_ovrd=off  block_type=constant
  Constant5 : xbsIndex_r4/Constant  const=h(6,11)  gui_display_data_type=Fixed-point  arith_type=Signed (2's comp)  n_bits=W  bin_pt=B  preci_type=Single  exp_width=8  frac_width=24  explicit_period=off  period=1  equ=P=C  opselect=C  inp2=PCIN>>17  opr=+  inp1=P  carry=CIN  dbl_ovrd=off  block_type=constant
  Constant6 : xbsIndex_r4/Constant  const=h(7,11)  gui_display_data_type=Fixed-point  arith_type=Signed (2's comp)  n_bits=W  bin_pt=B  preci_type=Single  exp_width=8  frac_width=24  explicit_period=off  period=1  equ=P=C  opselect=C  inp2=PCIN>>17  opr=+  inp1=P  carry=CIN  dbl_ovrd=off  block_type=constant
  Constant7 : xbsIndex_r4/Constant  const=h(8,11)  gui_display_data_type=Fixed-point  arith_type=Signed (2's comp)  n_bits=W  bin_pt=B  preci_type=Single  exp_width=8  frac_width=24  explicit_period=off  period=1  equ=P=C  opselect=C  inp2=PCIN>>17  opr=+  inp1=P  carry=CIN  dbl_ovrd=off  block_type=constant
  Constant8 : xbsIndex_r4/Constant  const=h(9,11)  gui_display_data_type=Fixed-point  arith_type=Signed (2's comp)  n_bits=W  bin_pt=B  preci_type=Single  exp_width=8  frac_width=24  explicit_period=off  period=1  equ=P=C  opselect=C  inp2=PCIN>>17  opr=+  inp1=P  carry=CIN  dbl_ovrd=off  block_type=constant
  Constant9 : xbsIndex_r4/Constant  const=h(10,11)  gui_display_data_type=Fixed-point  arith_type=Signed (2's comp)  n_bits=W  bin_pt=B  preci_type=Single  exp_width=8  frac_width=24  explicit_period=off  period=1  equ=P=C  opselect=C  inp2=PCIN>>17  opr=+  inp1=P  carry=CIN  dbl_ovrd=off  block_type=constant
  Delay{1..32} (32 alike) : xbsIndex_r4/Delay  rst=off  infoeditControl=Selection of Reset will increase slice count due to use of real FFs and instead of SRLs  en=off  latency=1  reg_retiming=off  dbl_ovrd=off  block_type=delay
  Mult{,15..30} (17 alike) : xbsIndex_r4/Mult  precision=User Defined  arith_type="Signed  (2's comp)"  n_bits=W  bin_pt=B  quantization="Round  (unbiased: +/- Inf)"  overflow=Flag as error  en=off  latency=0  use_behavioral_HDL=off  opt=Speed  use_embedded=on  optimum_pipeline=off  pipeline=on  dbl_ovrd=off  use_rpm=on  placement_style=Triangular  block_type=mult
  Out1 : Outport
  wires:
  AddSub2/1 -> Out1/1
  Constant14/1 -> Mult16/2
  Mult/1 -> AddSub16/2
  Mult16/1 -> AddSub1/2
  Constant15/1 -> Mult/2
  Constant13/1 -> Mult17/2
  Mult17/1 -> AddSub18/2
  Constant12/1 -> Mult18/2
  Constant11/1 -> Mult19/2
  Mult19/1 -> AddSub20/2
  Constant10/1 -> Mult20/2
  Mult20/1 -> AddSub19/2
  Constant9/1 -> Mult21/2
  Mult21/1 -> AddSub22/2
  Constant8/1 -> Mult22/2
  Constant7/1 -> Mult23/2
  Mult23/1 -> AddSub24/2
  Constant6/1 -> Mult24/2
  Constant5/1 -> Mult25/2
  Mult25/1 -> AddSub26/2
  Constant4/1 -> Mult26/2
  Mult26/1 -> AddSub25/2
  Constant3/1 -> Mult27/2
  Mult27/1 -> AddSub28/2
  Constant2/1 -> Mult28/2
  Constant1/1 -> Mult29/2
  Mult29/1 -> AddSub30/2
  Constant/1 -> Mult30/2
  AddSub1/1 -> AddSub16/1
  AddSub18/1 -> AddSub1/1
  AddSub17/1 -> AddSub18/1
  AddSub19/1 -> AddSub20/1
  AddSub22/1 -> AddSub19/1
  AddSub21/1 -> AddSub22/1
  AddSub23/1 -> AddSub24/1
  AddSub25/1 -> AddSub26/1
  AddSub28/1 -> AddSub25/1
  AddSub27/1 -> AddSub28/1
  Mult30/1 -> AddSub30/1
  Constant16/1 -> Mult15/2
  Mult15/1 -> AddSub2/2
  AddSub16/1 -> AddSub2/1
  AddSub20/1 -> AddSub17/1
  Mult18/1 -> AddSub17/2
  AddSub24/1 -> AddSub21/1
  Mult22/1 -> AddSub21/2
  AddSub26/1 -> AddSub23/1
  Mult24/1 -> AddSub23/2
  AddSub30/1 -> AddSub27/1
  Mult28/1 -> AddSub27/2
  In1/1 -> AddSub3/1, Delay1/1
  Delay1/1 -> AddSub4/1, Delay15/1
  Delay15/1 -> AddSub5/1, Delay2/1
  Delay2/1 -> AddSub6/1, Delay3/1
  Delay3/1 -> AddSub7/1, Delay4/1
  Delay4/1 -> AddSub8/1, Delay5/1
  Delay5/1 -> AddSub9/1, Delay6/1
  Delay6/1 -> AddSub10/1, Delay7/1
  Delay7/1 -> AddSub11/1, Delay8/1
  Delay8/1 -> AddSub12/1, Delay9/1
  Delay9/1 -> AddSub13/1, Delay10/1
  Delay10/1 -> AddSub14/1, Delay11/1
  Delay11/1 -> AddSub15/1, Delay12/1
  Delay12/1 -> AddSub29/1, Delay13/1
  Delay13/1 -> AddSub31/1, Delay14/1
  Delay14/1 -> AddSub32/1, Delay16/1
  In2/1 -> AddSub33/2, Delay17/1
  Delay17/1 -> AddSub32/2, Delay23/1
  Delay23/1 -> AddSub31/2, Delay25/1
  Delay25/1 -> AddSub29/2, Delay26/1
  Delay26/1 -> AddSub15/2, Delay27/1
  Delay27/1 -> AddSub14/2, Delay28/1
  Delay28/1 -> AddSub13/2, Delay29/1
  Delay29/1 -> AddSub12/2, Delay30/1
  Delay30/1 -> AddSub11/2, Delay31/1
  Delay31/1 -> AddSub10/2, Delay32/1
  Delay32/1 -> AddSub9/2, Delay18/1
  Delay18/1 -> AddSub8/2, Delay19/1
  Delay19/1 -> AddSub7/2, Delay20/1
  Delay20/1 -> AddSub6/2, Delay21/1
  Delay21/1 -> AddSub5/2, Delay22/1
  Delay22/1 -> AddSub4/2, Delay24/1
  AddSub3/1 -> Mult30/1
  Delay16/1 -> AddSub33/1
  AddSub33/1 -> Mult15/1
  AddSub32/1 -> Mult/1
  AddSub31/1 -> Mult16/1
  AddSub29/1 -> Mult17/1
  AddSub15/1 -> Mult18/1
  AddSub14/1 -> Mult19/1
  AddSub13/1 -> Mult20/1
  AddSub12/1 -> Mult21/1
  AddSub11/1 -> Mult22/1
  AddSub10/1 -> Mult23/1
  AddSub9/1 -> Mult24/1
  AddSub8/1 -> Mult25/1
  AddSub7/1 -> Mult26/1
  AddSub6/1 -> Mult27/1
  AddSub5/1 -> Mult28/1
  AddSub4/1 -> Mult29/1
  Delay24/1 -> AddSub3/2

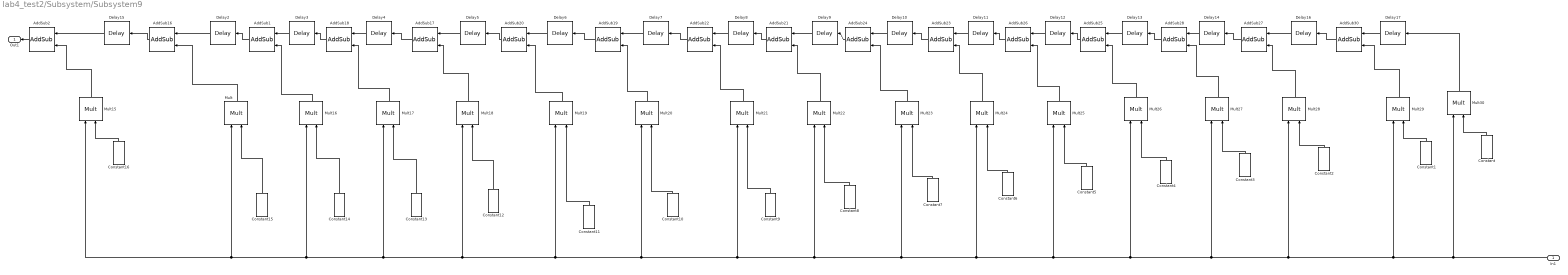
== system lab4_test2/Subsystem/Subsystem9 ==
  In1 : Inport
  AddSub{1..2,16..28,30} (16 alike) : xbsIndex_r4/AddSub  mode=Addition  use_carryin=off  use_carryout=off  en=off  latency=0  precision=User Defined  arith_type="Signed  (2's comp)"  n_bits=W  bin_pt=B  quantization=Truncate  overflow=Wrap  use_behavioral_HDL=off  hw_selection=Fabric  pipelined=off  dbl_ovrd=off  block_type=addsub
  Constant : xbsIndex_r4/Constant  const=h(1,9)  gui_display_data_type=Fixed-point  arith_type=Signed (2's comp)  n_bits=W  bin_pt=B  preci_type=Single  exp_width=8  frac_width=24  explicit_period=off  period=1  equ=P=C  opselect=C  inp2=PCIN>>17  opr=+  inp1=P  carry=CIN  dbl_ovrd=off  block_type=constant
  Constant1 : xbsIndex_r4/Constant  const=h(2,9)  gui_display_data_type=Fixed-point  arith_type=Signed (2's comp)  n_bits=W  bin_pt=B  preci_type=Single  exp_width=8  frac_width=24  explicit_period=off  period=1  equ=P=C  opselect=C  inp2=PCIN>>17  opr=+  inp1=P  carry=CIN  dbl_ovrd=off  block_type=constant
  Constant10 : xbsIndex_r4/Constant  const=h(11,9)  gui_display_data_type=Fixed-point  arith_type=Signed (2's comp)  n_bits=W  bin_pt=B  preci_type=Single  exp_width=8  frac_width=24  explicit_period=off  period=1  equ=P=C  opselect=C  inp2=PCIN>>17  opr=+  inp1=P  carry=CIN  dbl_ovrd=off  block_type=constant
  Constant11 : xbsIndex_r4/Constant  const=h(12,9)  gui_display_data_type=Fixed-point  arith_type=Signed (2's comp)  n_bits=W  bin_pt=B  preci_type=Single  exp_width=8  frac_width=24  explicit_period=off  period=1  equ=P=C  opselect=C  inp2=PCIN>>17  opr=+  inp1=P  carry=CIN  dbl_ovrd=off  block_type=constant
  Constant12 : xbsIndex_r4/Constant  const=h(13,9)  gui_display_data_type=Fixed-point  arith_type=Signed (2's comp)  n_bits=W  bin_pt=B  preci_type=Single  exp_width=8  frac_width=24  explicit_period=off  period=1  equ=P=C  opselect=C  inp2=PCIN>>17  opr=+  inp1=P  carry=CIN  dbl_ovrd=off  block_type=constant
  Constant13 : xbsIndex_r4/Constant  const=h(14,9)  gui_display_data_type=Fixed-point  arith_type=Signed (2's comp)  n_bits=W  bin_pt=B  preci_type=Single  exp_width=8  frac_width=24  explicit_period=off  period=1  equ=P=C  opselect=C  inp2=PCIN>>17  opr=+  inp1=P  carry=CIN  dbl_ovrd=off  block_type=constant
  Constant14 : xbsIndex_r4/Constant  const=h(15,9)  gui_display_data_type=Fixed-point  arith_type=Signed (2's comp)  n_bits=W  bin_pt=B  preci_type=Single  exp_width=8  frac_width=24  explicit_period=off  period=1  equ=P=C  opselect=C  inp2=PCIN>>17  opr=+  inp1=P  carry=CIN  dbl_ovrd=off  block_type=constant
  Constant15 : xbsIndex_r4/Constant  const=h(16,9)  gui_display_data_type=Fixed-point  arith_type=Signed (2's comp)  n_bits=W  bin_pt=B  preci_type=Single  exp_width=8  frac_width=24  explicit_period=off  period=1  equ=P=C  opselect=C  inp2=PCIN>>17  opr=+  inp1=P  carry=CIN  dbl_ovrd=off  block_type=constant
  Constant16 : xbsIndex_r4/Constant  const=h(17,9)  gui_display_data_type=Fixed-point  arith_type=Signed (2's comp)  n_bits=W  bin_pt=B  preci_type=Single  exp_width=8  frac_width=24  explicit_period=off  period=1  equ=P=C  opselect=C  inp2=PCIN>>17  opr=+  inp1=P  carry=CIN  dbl_ovrd=off  block_type=constant
  Constant2 : xbsIndex_r4/Constant  const=h(3,9)  gui_display_data_type=Fixed-point  arith_type=Signed (2's comp)  n_bits=W  bin_pt=B  preci_type=Single  exp_width=8  frac_width=24  explicit_period=off  period=1  equ=P=C  opselect=C  inp2=PCIN>>17  opr=+  inp1=P  carry=CIN  dbl_ovrd=off  block_type=constant
  Constant3 : xbsIndex_r4/Constant  const=h(4,9)  gui_display_data_type=Fixed-point  arith_type=Signed (2's comp)  n_bits=W  bin_pt=B  preci_type=Single  exp_width=8  frac_width=24  explicit_period=off  period=1  equ=P=C  opselect=C  inp2=PCIN>>17  opr=+  inp1=P  carry=CIN  dbl_ovrd=off  block_type=constant
  Constant4 : xbsIndex_r4/Constant  const=h(5,9)  gui_display_data_type=Fixed-point  arith_type=Signed (2's comp)  n_bits=W  bin_pt=B  preci_type=Single  exp_width=8  frac_width=24  explicit_period=off  period=1  equ=P=C  opselect=C  inp2=PCIN>>17  opr=+  inp1=P  carry=CIN  dbl_ovrd=off  block_type=constant
  Constant5 : xbsIndex_r4/Constant  const=h(6,9)  gui_display_data_type=Fixed-point  arith_type=Signed (2's comp)  n_bits=W  bin_pt=B  preci_type=Single  exp_width=8  frac_width=24  explicit_period=off  period=1  equ=P=C  opselect=C  inp2=PCIN>>17  opr=+  inp1=P  carry=CIN  dbl_ovrd=off  block_type=constant
  Constant6 : xbsIndex_r4/Constant  const=h(7,9)  gui_display_data_type=Fixed-point  arith_type=Signed (2's comp)  n_bits=W  bin_pt=B  preci_type=Single  exp_width=8  frac_width=24  explicit_period=off  period=1  equ=P=C  opselect=C  inp2=PCIN>>17  opr=+  inp1=P  carry=CIN  dbl_ovrd=off  block_type=constant
  Constant7 : xbsIndex_r4/Constant  const=h(8,9)  gui_display_data_type=Fixed-point  arith_type=Signed (2's comp)  n_bits=W  bin_pt=B  preci_type=Single  exp_width=8  frac_width=24  explicit_period=off  period=1  equ=P=C  opselect=C  inp2=PCIN>>17  opr=+  inp1=P  carry=CIN  dbl_ovrd=off  block_type=constant
  Constant8 : xbsIndex_r4/Constant  const=h(9,9)  gui_display_data_type=Fixed-point  arith_type=Signed (2's comp)  n_bits=W  bin_pt=B  preci_type=Single  exp_width=8  frac_width=24  explicit_period=off  period=1  equ=P=C  opselect=C  inp2=PCIN>>17  opr=+  inp1=P  carry=CIN  dbl_ovrd=off  block_type=constant
  Constant9 : xbsIndex_r4/Constant  const=h(10,9)  gui_display_data_type=Fixed-point  arith_type=Signed (2's comp)  n_bits=W  bin_pt=B  preci_type=Single  exp_width=8  frac_width=24  explicit_period=off  period=1  equ=P=C  opselect=C  inp2=PCIN>>17  opr=+  inp1=P  carry=CIN  dbl_ovrd=off  block_type=constant
  Delay{2..17} (16 alike) : xbsIndex_r4/Delay  rst=off  infoeditControl=Selection of Reset will increase slice count due to use of real FFs and instead of SRLs  en=off  latency=1  reg_retiming=off  dbl_ovrd=off  block_type=delay
  Mult{,15..30} (17 alike) : xbsIndex_r4/Mult  precision=User Defined  arith_type="Signed  (2's comp)"  n_bits=W  bin_pt=B  quantization="Round  (unbiased: +/- Inf)"  overflow=Flag as error  en=off  latency=0  use_behavioral_HDL=off  opt=Speed  use_embedded=on  optimum_pipeline=off  pipeline=on  dbl_ovrd=off  use_rpm=on  placement_style=Triangular  block_type=mult
  Out1 : Outport
  wires:
  AddSub2/1 -> Out1/1
  Constant14/1 -> Mult16/2
  Mult/1 -> AddSub16/2
  Mult16/1 -> AddSub1/2
  AddSub16/1 -> Delay15/1
  Constant15/1 -> Mult/2
  AddSub1/1 -> Delay2/1
  Constant13/1 -> Mult17/2
  Mult17/1 -> AddSub18/2
  Constant12/1 -> Mult18/2
  AddSub17/1 -> Delay4/1
  AddSub18/1 -> Delay3/1
  Constant11/1 -> Mult19/2
  Mult19/1 -> AddSub20/2
  Constant10/1 -> Mult20/2
  Mult20/1 -> AddSub19/2
  AddSub19/1 -> Delay6/1
  AddSub20/1 -> Delay5/1
  Constant9/1 -> Mult21/2
  Mult21/1 -> AddSub22/2
  Constant8/1 -> Mult22/2
  AddSub21/1 -> Delay8/1
  AddSub22/1 -> Delay7/1
  Constant7/1 -> Mult23/2
  Mult23/1 -> AddSub24/2
  Constant6/1 -> Mult24/2
  AddSub23/1 -> Delay10/1
  Constant5/1 -> Mult25/2
  Mult25/1 -> AddSub26/2
  Constant4/1 -> Mult26/2
  Mult26/1 -> AddSub25/2
  AddSub25/1 -> Delay12/1
  AddSub26/1 -> Delay11/1
  Constant3/1 -> Mult27/2
  Mult27/1 -> AddSub28/2
  Constant2/1 -> Mult28/2
  AddSub27/1 -> Delay14/1
  AddSub28/1 -> Delay13/1
  Constant1/1 -> Mult29/2
  Mult29/1 -> AddSub30/2
  Constant/1 -> Mult30/2
  Mult30/1 -> Delay17/1
  AddSub30/1 -> Delay16/1
  AddSub24/1 -> Delay9/1
  Delay2/1 -> AddSub16/1
  Delay3/1 -> AddSub1/1
  Delay4/1 -> AddSub18/1
  Delay6/1 -> AddSub20/1
  Delay7/1 -> AddSub19/1
  Delay8/1 -> AddSub22/1
  Delay10/1 -> AddSub24/1
  Delay12/1 -> AddSub26/1
  Delay13/1 -> AddSub25/1
  Delay14/1 -> AddSub28/1
  Delay17/1 -> AddSub30/1
  Constant16/1 -> Mult15/2
  Mult15/1 -> AddSub2/2
  Delay15/1 -> AddSub2/1
  Delay5/1 -> AddSub17/1
  Mult18/1 -> AddSub17/2
  Delay9/1 -> AddSub21/1
  Mult22/1 -> AddSub21/2
  Delay11/1 -> AddSub23/1
  Mult24/1 -> AddSub23/2
  Delay16/1 -> AddSub27/1
  Mult28/1 -> AddSub27/2
  In1/1 -> Mult30/1, Mult29/1, Mult28/1, Mult27/1, Mult26/1, Mult25/1, Mult24/1, Mult22/1, Mult21/1, Mult19/1, Mult17/1, Mult15/1, Mult/1, Mult16/1, Mult18/1, Mult20/1, Mult23/1
